simulink model "FullCarModelSim"  (R2018a)
settings: Solver=VariableStepAuto  StartTime=0.0  StopTime=8  FixedStep=0.001  MaxStep=0.002  MinStep=0.001  RelTol=1e-3  EnableMultiTasking=on
undefined symbols (not defined in the file): a, b, cg_height, cla, cp, I_zz, LLTD, m, step_steer, track_width_f, track_width_r, weight_dist, X
settings Model: Creator=tonylu  LastModifiedBy=tlton
settings OptimizationCC: LifeSpan=inf
settings DebuggingCC: SFUnexpectedBacktrackingDiag=warning  SFNoUnconditionalDefaultTransitionDiag=warning  SFExecutionAtInitializationDiag=none
settings CodeAppCC: StateflowObjectComments=on
settings GRTTargetCC: TargetLangStandard=C89/C90 (ANSI)  GeneratePreprocessorConditionals=Disable all
settings ConfigComp: CovMetricSettings=dw  CovHtmlReporting=on  CovSaveCumulativeToWorkspaceVar=on  CovSaveSingleToWorkspaceVar=on  CovExternalEMLEnable=off

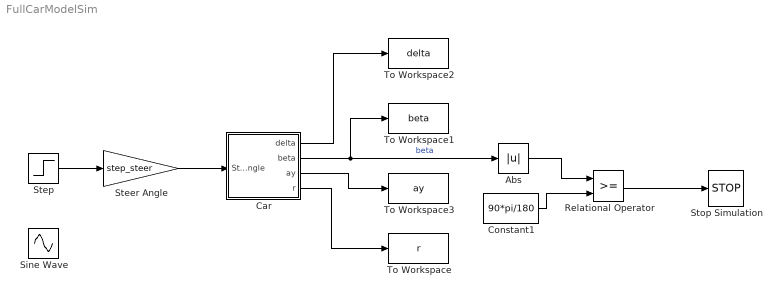
== system FullCarModelSim ==
  Abs : Abs
  Car : Subsystem
  Constant1 : Constant  Value=90*pi/180
  Relational Operator : RelationalOperator  OutDataTypeStr=boolean  RndMeth=Simplest
  Sine Wave : Sin  SampleTime=0
  Steer Angle : Gain  Gain=step_steer
  Step : Step  Time=0  SampleTime=0
  Stop Simulation : Stop
  To Workspace : ToWorkspace  VariableName=r  SaveFormat=Structure With Time  SampleTime=0.01
  To Workspace1 : ToWorkspace  VariableName=beta  SaveFormat=Structure With Time  SampleTime=0.01
  To Workspace2 : ToWorkspace  VariableName=delta  SaveFormat=Structure With Time  SampleTime=0.01
  To Workspace3 : ToWorkspace  VariableName=ay  SaveFormat=Structure With Time  SampleTime=0.01
  wires:
  Car/1(delta) -> To Workspace2/1
  Car/3(ay) -> To Workspace3/1
  Car/4(r) -> To Workspace/1
  Steer Angle/1 -> Car/1(Steer Angle)
  Car/2(beta) -> Abs/1, To Workspace1/1  "beta"
  Relational Operator/1 -> Stop Simulation/1
  Constant1/1 -> Relational Operator/2
  Abs/1 -> Relational Operator/1
  Step/1 -> Steer Angle/1

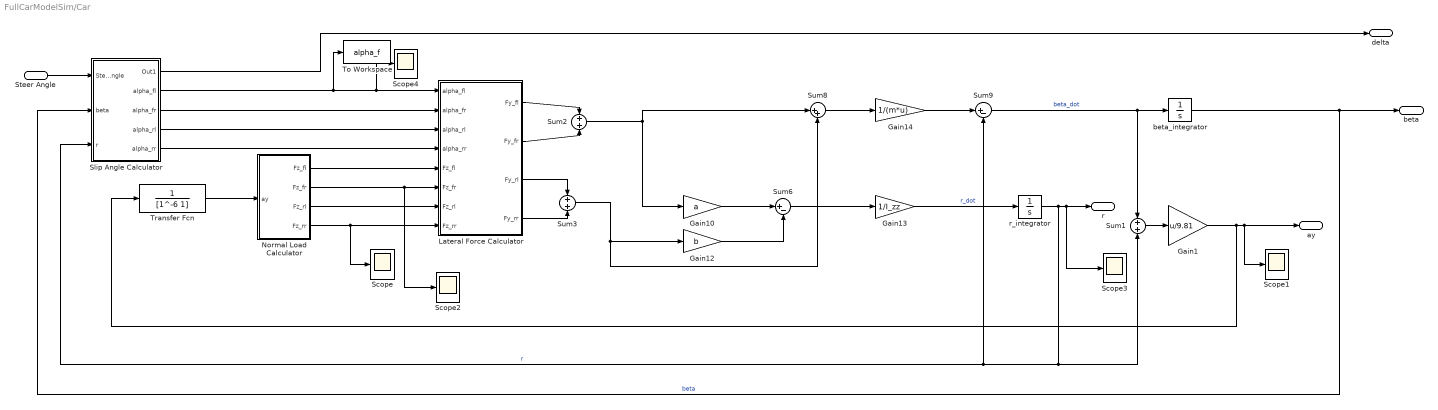
== system FullCarModelSim/Car ==
  Steer Angle : Inport
  Gain1 : Gain  Gain=u/9.81
  Gain10 : Gain  Gain=a
  Gain12 : Gain  Gain=b
  Gain13 : Gain  Gain=1/I_zz
  Gain14 : Gain  Gain=1/(m*u)
  Lateral Force Calculator : Subsystem
  Normal Load Calculator : Subsystem
  Scope{,1..4} (5 alike) : Scope
  Slip Angle Calculator : Subsystem
  Sum1 : Sum  Inputs=+|+
  Sum2 : Sum  Inputs=+|+
  Sum3 : Sum  Inputs=+|+
  Sum6 : Sum  Inputs=|+-
  Sum8 : Sum  Inputs=|++
  Sum9 : Sum  Inputs=|+-
  To Workspace : ToWorkspace  VariableName=alpha_f  SaveFormat=Structure With Time  SampleTime=0.01
  Transfer Fcn : TransferFcn  Denominator=[1^-6 1]
  beta_integrator : Integrator
  r_integrator : Integrator
  delta : Outport
  beta : Outport  Port=2
  ay : Outport  Port=3
  r : Outport  Port=4
  wires:
  Gain10/1 -> Sum6/1
  Gain12/1 -> Sum6/2
  Sum6/1 -> Gain13/1
  Gain13/1 -> r_integrator/1  "r_dot"
  Sum8/1 -> Gain14/1
  Gain14/1 -> Sum9/1
  Sum1/1 -> Gain1/1
  Steer Angle/1 -> Slip Angle Calculator/1(Steer Angle)
  Slip Angle Calculator/1(Out1) -> delta/1
  Slip Angle Calculator/2(alpha_fl) -> To Workspace/1, Scope4/1, Lateral Force Calculator/1(alpha_fl)
  Slip Angle Calculator/3(alpha_fr) -> Lateral Force Calculator/2(alpha_fr)
  Sum9/1 -> beta_integrator/1, Sum1/1  "beta_dot"
  beta_integrator/1 -> beta/1, Slip Angle Calculator/2(beta)  "beta"
  r_integrator/1 -> Slip Angle Calculator/3(r), Sum9/2, Sum1/2, Scope3/1, r/1  "r"
  Slip Angle Calculator/4(alpha_rl) -> Lateral Force Calculator/3(alpha_rl)
  Slip Angle Calculator/5(alpha_rr) -> Lateral Force Calculator/4(alpha_rr)
  Normal Load Calculator/1(Fz_fl) -> Lateral Force Calculator/5(Fz_fl)
  Normal Load Calculator/3(Fz_rl) -> Lateral Force Calculator/7(Fz_rl)
  Lateral Force Calculator/2(Fy_fr) -> Sum2/2
  Lateral Force Calculator/1(Fy_fl) -> Sum2/1
  Sum2/1 -> Gain10/1, Sum8/1
  Lateral Force Calculator/3(Fy_rl) -> Sum3/1
  Lateral Force Calculator/4(Fy_rr) -> Sum3/2
  Sum3/1 -> Sum8/2, Gain12/1
  Gain1/1 -> Transfer Fcn/1, Scope1/1, ay/1
  Normal Load Calculator/4("Fz_rr ") -> Scope/1, Lateral Force Calculator/8(Fz_rr)
  Normal Load Calculator/2(Fz_fr) -> Scope2/1, Lateral Force Calculator/6(Fz_fr)
  Transfer Fcn/1 -> Normal Load Calculator/1(ay)

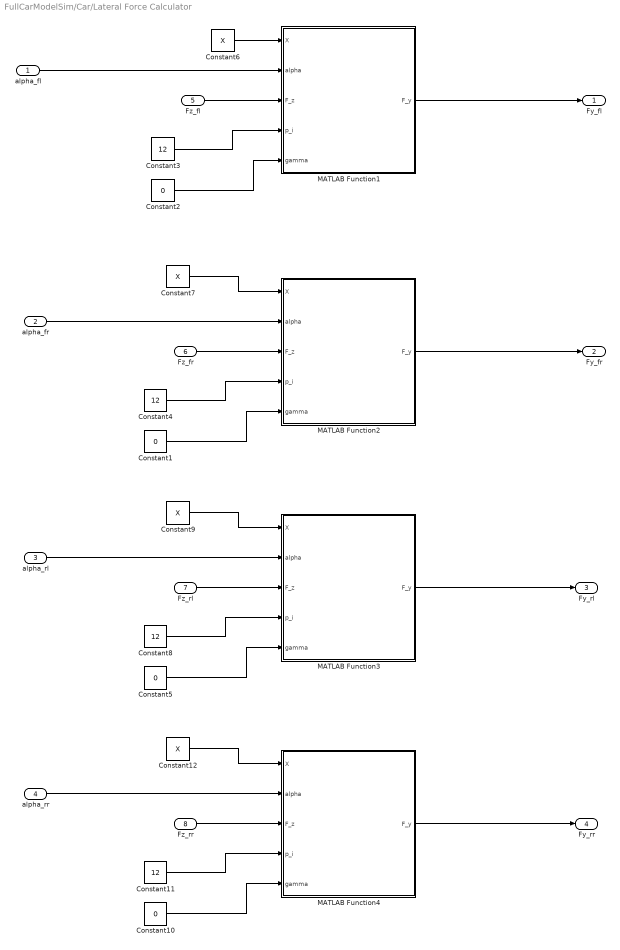
== system FullCarModelSim/Car/Lateral Force Calculator ==
  alpha_fl : Inport
  alpha_fr : Inport  Port=2
  alpha_rl : Inport  Port=3
  alpha_rr : Inport  Port=4
  Fz_fl : Inport  Port=5
  Fz_fr : Inport  Port=6
  Fz_rl : Inport  Port=7
  Fz_rr : Inport  Port=8
  Constant{1..2,5,10} (4 alike) : Constant  Value=0
  Constant{3..4,8,11} (4 alike) : Constant  Value=12
  Constant{6..7,9,12} (4 alike) : Constant  Value=X
  MATLAB Function1 : MATLAB Function  TreatAsAtomicUnit=on
  MATLAB Function2 : MATLAB Function  TreatAsAtomicUnit=on
  MATLAB Function3 : MATLAB Function  TreatAsAtomicUnit=on
  MATLAB Function4 : MATLAB Function  TreatAsAtomicUnit=on
  Fy_fl : Outport
  Fy_fr : Outport  Port=2
  Fy_rl : Outport  Port=3
  Fy_rr : Outport  Port=4
  wires:
  MATLAB Function2/1(F_y) -> Fy_fr/1
  Fz_fl/1 -> MATLAB Function1/3(F_z)
  Constant3/1 -> MATLAB Function1/4(p_i)
  Fz_fr/1 -> MATLAB Function2/3(F_z)
  MATLAB Function1/1(F_y) -> Fy_fl/1
  alpha_fr/1 -> MATLAB Function2/2(alpha)
  alpha_fl/1 -> MATLAB Function1/2(alpha)
  Constant4/1 -> MATLAB Function2/4(p_i)
  Constant2/1 -> MATLAB Function1/5(gamma)
  Constant7/1 -> MATLAB Function2/1(X)
  Constant6/1 -> MATLAB Function1/1(X)
  Constant1/1 -> MATLAB Function2/5(gamma)
  MATLAB Function3/1(F_y) -> Fy_rl/1
  Constant5/1 -> MATLAB Function3/5(gamma)
  alpha_rl/1 -> MATLAB Function3/2(alpha)
  Constant9/1 -> MATLAB Function3/1(X)
  Constant8/1 -> MATLAB Function3/4(p_i)
  Fz_rl/1 -> MATLAB Function3/3(F_z)
  MATLAB Function4/1(F_y) -> Fy_rr/1
  Constant10/1 -> MATLAB Function4/5(gamma)
  alpha_rr/1 -> MATLAB Function4/2(alpha)
  Constant12/1 -> MATLAB Function4/1(X)
  Constant11/1 -> MATLAB Function4/4(p_i)
  Fz_rr/1 -> MATLAB Function4/3(F_z)

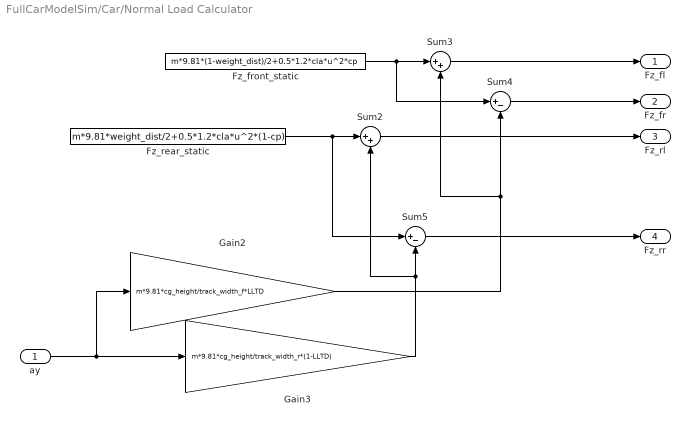
== system FullCarModelSim/Car/Normal Load Calculator ==
  ay : Inport
  Fz_front_static : Constant  Value=m*9.81*(1-weight_dist)/2+0.5*1.2*cla*u^2*cp
  Fz_rear_static : Constant  Value=m*9.81*weight_dist/2+0.5*1.2*cla*u^2*(1-cp)
  Gain2 : Gain  Gain=m*9.81*cg_height/track_width_f*LLTD
  Gain3 : Gain  Gain=m*9.81*cg_height/track_width_r*(1-LLTD)
  Sum2 : Sum  Inputs=|++
  Sum3 : Sum  Inputs=|++
  Sum4 : Sum  Inputs=|+-
  Sum5 : Sum  Inputs=|+-
  Fz_fl : Outport
  Fz_fr : Outport  Port=2
  Fz_rl : Outport  Port=3
  "Fz_rr " : Outport  Port=4
  wires:
  Sum4/1 -> Fz_fr/1
  Sum5/1 -> "Fz_rr "/1
  Fz_front_static/1 -> Sum4/1, Sum3/1
  Fz_rear_static/1 -> Sum5/1, Sum2/1
  Sum2/1 -> Fz_rl/1
  Gain3/1 -> Sum2/2, Sum5/2
  Sum3/1 -> Fz_fl/1
  ay/1 -> Gain2/1, Gain3/1
  Gain2/1 -> Sum4/2, Sum3/2

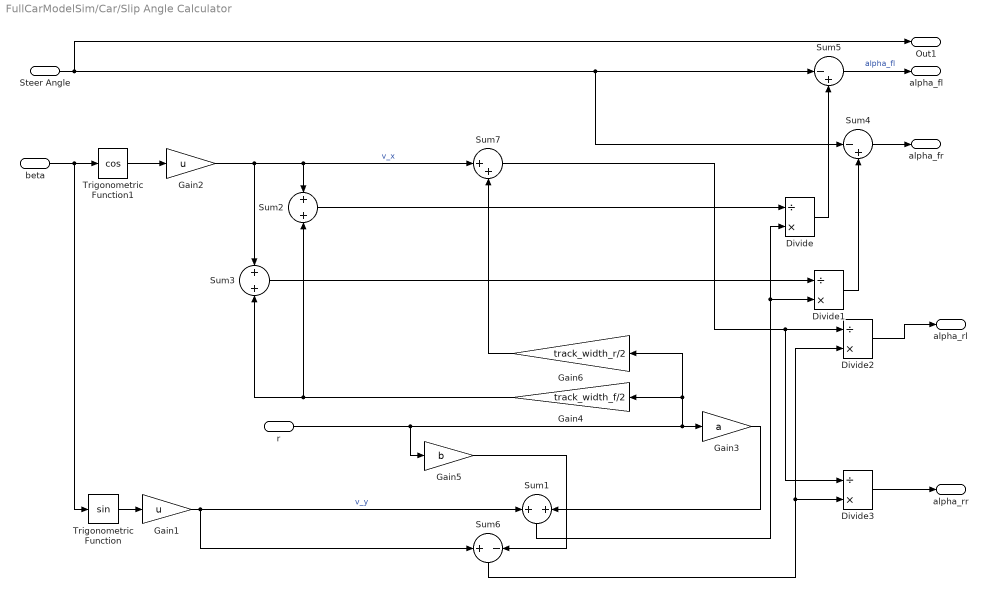
== system FullCarModelSim/Car/Slip Angle Calculator ==
  Steer Angle : Inport
  beta : Inport  Port=2
  r : Inport  Port=3
  Divide{,1..3} (4 alike) : Product  Inputs=/*
  Gain1 : Gain  Gain=u
  Gain2 : Gain  Gain=u
  Gain3 : Gain  Gain=a
  Gain4 : Gain  Gain=track_width_f/2
  Gain5 : Gain  Gain=b
  Gain6 : Gain  Gain=track_width_r/2
  Sum1 : Sum  Inputs=+|+
  Sum2 : Sum  Inputs=+|+
  Sum3 : Sum  Inputs=+|+
  Sum4 : Sum  Inputs=|-+
  Sum5 : Sum  Inputs=|-+
  Sum6 : Sum  Inputs=+|-
  Sum7 : Sum  Inputs=|++
  Trigonometric Function : Trigonometry
  Trigonometric Function1 : Trigonometry  Operator=cos
  Out1 : Outport
  alpha_fl : Outport  Port=2
  alpha_fr : Outport  Port=3
  alpha_rl : Outport  Port=4
  alpha_rr : Outport  Port=5
  wires:
  Sum5/1 -> alpha_fl/1  "alpha_fl"
  Trigonometric Function/1 -> Gain1/1
  Gain3/1 -> Sum1/2
  Divide/1 -> Sum5/2
  Sum3/1 -> Divide1/1
  Divide1/1 -> Sum4/2
  Sum4/1 -> alpha_fr/1
  Gain5/1 -> Sum6/2
  Sum2/1 -> Divide/1
  Divide2/1 -> alpha_rl/1
  Gain6/1 -> Sum7/2
  Divide3/1 -> alpha_rr/1
  Sum7/1 -> Divide3/1, Divide2/1
  Sum6/1 -> Divide3/2, Divide2/2
  Gain4/1 -> Sum3/2, Sum2/2
  Sum1/1 -> Divide1/2, Divide/2
  Gain1/1 -> Sum6/1, Sum1/1  "v_y"
  Gain2/1 -> Sum7/1, Sum2/1, Sum3/1  "v_x"
  Steer Angle/1 -> Sum4/1, Sum5/1, Out1/1
  r/1 -> Gain5/1, Gain6/1, Gain4/1, Gain3/1
  Trigonometric Function1/1 -> Gain2/1
  beta/1 -> Trigonometric Function/1, Trigonometric Function1/1

== matlab function FullCarModelSim/Car/Lateral Force Calculator/MATLAB Function1 ==
  data: X input; F_y output; alpha input; F_z input; p_i input; gamma input
function F_y  = lateralforce_pure(X,alpha,F_z,p_i,gamma)
%% Inputs
F_z = F_z/4.44822; % N to lbf

F_z0 = 200*ones(size(F_z)); %nominal load
p_i0 = 13*ones(size(p_i)); %nominal pressure

F_z = abs(F_z);

df_z = (F_z- F_z0)./F_z;
dp_i = (p_i-p_i0)./p_i;

%% Parameters

p_cy1 = X(1);
p_dy1 = X(2);
p_dy2 = X(3);
p_dy3 = X(4);
p_ey1 = X(5);
p_ey2 = X(6);
p_ey3 = X(7);
p_ey4 = X(8);
p_ey5 = X(9);
p_hy1 = X(10);
p_hy2 = X(11);
p_ky1 = X(12);
p_ky2 = X(13);
p_ky3 = X(14);
p_ky4 = X(15);
p_ky5 = X(16);
p_ky6 = X(17);
p_ky7 = X(18);
p_py1 = X(19);
p_py2 = X(20);
p_py3 = X(21);
p_py4 = X(22);
p_py5 = X(23);
p_vy1 = X(24);
p_vy2 = X(25);
p_vy3 = X(26);
p_vy4 = X(27);

%p_ey3 = 0
%p_dy1 = 1.8;
%p_dy2 = -0.05;

lambda_cy = 1;       % shape factor   
lambda_ey = 1;       % curvature 
lambda_hy = 0;       % horizontal shift
lambda_kyalpha = 1;  % cornering stiffness
lambda_kygamma = 1;  % camber force stiffness
lambda_muy = 0.55;      % peak friction coefficient
lambda_vy = 0;       % vertical shift

%%  Magic Formula Equations

K_yalpha = p_ky1.*F_z0.*(1+p_py1.*dp_i).*sin(p_ky4.*atan(F_z./...
    ((p_ky2 + p_ky5*gamma.^2).*(1+p_py2*dp_i).*F_z0))).*...
    (1-p_ky3.*abs(gamma)).*lambda_kyalpha;
K_ygamma = (p_ky6+p_ky7.*df_z).*(1+p_py5.*dp_i).*F_z.*lambda_kygamma;
S_vy0 = F_z.*(p_vy1+p_vy2.*df_z).*lambda_vy.*lambda_muy;
S_vygamma = F_z.*(p_vy3+p_vy4.*df_z).*gamma.*lambda_kygamma.*lambda_muy;
S_vy = S_vy0+S_vygamma;
S_hy0 = (p_hy1+p_hy2.*df_z).*lambda_hy;
S_hygamma = (K_ygamma.*gamma-S_vygamma)./K_yalpha;
S_hy = S_hy0+S_hygamma;
alpha_y = alpha+S_hy;
mu_y = (p_dy1+p_dy2.*df_z).*(1-p_dy3.*gamma.^2).*...
    (1+p_py3.*dp_i+p_py4.*dp_i.^2).*lambda_muy;
C_y = p_cy1.*lambda_cy;
D_y = mu_y.*F_z;
E_y = (p_ey1+p_ey2.*df_z).*(1+p_ey5.*gamma.^2-(p_ey3+p_ey4.*gamma).*sign(alpha_y)).*lambda_ey;
B_y = K_yalpha./C_y./D_y;

%Lateral Force
F_y = transpose(D_y.*sin(C_y.*atan(B_y.*alpha_y-E_y.*(B_y.*alpha_y-atan(B_y.*alpha_y))))+S_vy);

F_y = F_y*4.44822; % lbf to N

%F_y = -136*4.448*180/pi/2*alpha_y;

%F_y(F_z==0) = 0; %zero load

%F_y = K_yalpha*-0.0174533;

%F_y = -D_y

%F_y = mu_y;

end

== matlab function FullCarModelSim/Car/Lateral Force Calculator/MATLAB Function2 ==
  data: X input; F_y output; alpha input; F_z input; p_i input; gamma input
function F_y  = lateralforce_pure(X,alpha,F_z,p_i,gamma)
%% Inputs
F_z = F_z/4.44822; % N to lbf

F_z0 = 200*ones(size(F_z)); %nominal load
p_i0 = 13*ones(size(p_i)); %nominal pressure

F_z = abs(F_z);

df_z = (F_z- F_z0)./F_z;
dp_i = (p_i-p_i0)./p_i;

%% Parameters

p_cy1 = X(1);
p_dy1 = X(2);
p_dy2 = X(3);
p_dy3 = X(4);
p_ey1 = X(5);
p_ey2 = X(6);
p_ey3 = X(7);
p_ey4 = X(8);
p_ey5 = X(9);
p_hy1 = X(10);
p_hy2 = X(11);
p_ky1 = X(12);
p_ky2 = X(13);
p_ky3 = X(14);
p_ky4 = X(15);
p_ky5 = X(16);
p_ky6 = X(17);
p_ky7 = X(18);
p_py1 = X(19);
p_py2 = X(20);
p_py3 = X(21);
p_py4 = X(22);
p_py5 = X(23);
p_vy1 = X(24);
p_vy2 = X(25);
p_vy3 = X(26);
p_vy4 = X(27);

%p_ey3 = 0
%p_dy1 = 1.8;
%p_dy2 = -0.05;

lambda_cy = 1;       % shape factor   
lambda_ey = 1;       % curvature 
lambda_hy = 0;       % horizontal shift
lambda_kyalpha = 1;  % cornering stiffness
lambda_kygamma = 1;  % camber force stiffness
lambda_muy = 0.55;      % peak friction coefficient
lambda_vy = 0;       % vertical shift

%%  Magic Formula Equations

K_yalpha = p_ky1.*F_z0.*(1+p_py1.*dp_i).*sin(p_ky4.*atan(F_z./...
    ((p_ky2 + p_ky5*gamma.^2).*(1+p_py2*dp_i).*F_z0))).*...
    (1-p_ky3.*abs(gamma)).*lambda_kyalpha;
K_ygamma = (p_ky6+p_ky7.*df_z).*(1+p_py5.*dp_i).*F_z.*lambda_kygamma;
S_vy0 = F_z.*(p_vy1+p_vy2.*df_z).*lambda_vy.*lambda_muy;
S_vygamma = F_z.*(p_vy3+p_vy4.*df_z).*gamma.*lambda_kygamma.*lambda_muy;
S_vy = S_vy0+S_vygamma;
S_hy0 = (p_hy1+p_hy2.*df_z).*lambda_hy;
S_hygamma = (K_ygamma.*gamma-S_vygamma)./K_yalpha;
S_hy = S_hy0+S_hygamma;
alpha_y = alpha+S_hy;
mu_y = (p_dy1+p_dy2.*df_z).*(1-p_dy3.*gamma.^2).*...
    (1+p_py3.*dp_i+p_py4.*dp_i.^2).*lambda_muy;
C_y = p_cy1.*lambda_cy;
D_y = mu_y.*F_z;
E_y = (p_ey1+p_ey2.*df_z).*(1+p_ey5.*gamma.^2-(p_ey3+p_ey4.*gamma).*sign(alpha_y)).*lambda_ey;
B_y = K_yalpha./C_y./D_y;

%Lateral Force
F_y = transpose(D_y.*sin(C_y.*atan(B_y.*alpha_y-E_y.*(B_y.*alpha_y-atan(B_y.*alpha_y))))+S_vy);

F_y = F_y*4.44822; % lbf to N

%F_y = -136*4.448*180/pi/2*alpha_y;

%F_y(F_z==0) = 0; %zero load

%F_y = K_yalpha*-0.0174533;

%F_y = -D_y

%F_y = mu_y;

end

== matlab function FullCarModelSim/Car/Lateral Force Calculator/MATLAB Function3 ==
  data: X input; F_y output; alpha input; F_z input; p_i input; gamma input
function F_y  = lateralforce_pure(X,alpha,F_z,p_i,gamma)
%% Inputs
F_z = F_z/4.44822; % N to lbf

F_z0 = 200*ones(size(F_z)); %nominal load
p_i0 = 13*ones(size(p_i)); %nominal pressure

F_z = abs(F_z);

df_z = (F_z- F_z0)./F_z;
dp_i = (p_i-p_i0)./p_i;

%% Parameters

p_cy1 = X(1);
p_dy1 = X(2);
p_dy2 = X(3);
p_dy3 = X(4);
p_ey1 = X(5);
p_ey2 = X(6);
p_ey3 = X(7);
p_ey4 = X(8);
p_ey5 = X(9);
p_hy1 = X(10);
p_hy2 = X(11);
p_ky1 = X(12);
p_ky2 = X(13);
p_ky3 = X(14);
p_ky4 = X(15);
p_ky5 = X(16);
p_ky6 = X(17);
p_ky7 = X(18);
p_py1 = X(19);
p_py2 = X(20);
p_py3 = X(21);
p_py4 = X(22);
p_py5 = X(23);
p_vy1 = X(24);
p_vy2 = X(25);
p_vy3 = X(26);
p_vy4 = X(27);

%p_ey3 = 0
%p_dy1 = 1.8;
%p_dy2 = -0.05;

lambda_cy = 1;       % shape factor   
lambda_ey = 1;       % curvature 
lambda_hy = 0;       % horizontal shift
lambda_kyalpha = 1;  % cornering stiffness
lambda_kygamma = 1;  % camber force stiffness
lambda_muy = 0.55;      % peak friction coefficient
lambda_vy = 0;       % vertical shift

%%  Magic Formula Equations

K_yalpha = p_ky1.*F_z0.*(1+p_py1.*dp_i).*sin(p_ky4.*atan(F_z./...
    ((p_ky2 + p_ky5*gamma.^2).*(1+p_py2*dp_i).*F_z0))).*...
    (1-p_ky3.*abs(gamma)).*lambda_kyalpha;
K_ygamma = (p_ky6+p_ky7.*df_z).*(1+p_py5.*dp_i).*F_z.*lambda_kygamma;
S_vy0 = F_z.*(p_vy1+p_vy2.*df_z).*lambda_vy.*lambda_muy;
S_vygamma = F_z.*(p_vy3+p_vy4.*df_z).*gamma.*lambda_kygamma.*lambda_muy;
S_vy = S_vy0+S_vygamma;
S_hy0 = (p_hy1+p_hy2.*df_z).*lambda_hy;
S_hygamma = (K_ygamma.*gamma-S_vygamma)./K_yalpha;
S_hy = S_hy0+S_hygamma;
alpha_y = alpha+S_hy;
mu_y = (p_dy1+p_dy2.*df_z).*(1-p_dy3.*gamma.^2).*...
    (1+p_py3.*dp_i+p_py4.*dp_i.^2).*lambda_muy;
C_y = p_cy1.*lambda_cy;
D_y = mu_y.*F_z;
E_y = (p_ey1+p_ey2.*df_z).*(1+p_ey5.*gamma.^2-(p_ey3+p_ey4.*gamma).*sign(alpha_y)).*lambda_ey;
B_y = K_yalpha./C_y./D_y;

%Lateral Force
F_y = transpose(D_y.*sin(C_y.*atan(B_y.*alpha_y-E_y.*(B_y.*alpha_y-atan(B_y.*alpha_y))))+S_vy);

F_y = F_y*4.44822; % lbf to N

%F_y = -136*4.448*180/pi/2*alpha_y;

%F_y(F_z==0) = 0; %zero load

%F_y = K_yalpha*-0.0174533;

%F_y = -D_y

%F_y = mu_y;

end

== matlab function FullCarModelSim/Car/Lateral Force Calculator/MATLAB Function4 ==
  data: X input; F_y output; alpha input; F_z input; p_i input; gamma input
function F_y  = lateralforce_pure(X,alpha,F_z,p_i,gamma)
%% Inputs
F_z = F_z/4.44822; % N to lbf

F_z0 = 200*ones(size(F_z)); %nominal load
p_i0 = 13*ones(size(p_i)); %nominal pressure

F_z = abs(F_z);

df_z = (F_z- F_z0)./F_z;
dp_i = (p_i-p_i0)./p_i;

%% Parameters

p_cy1 = X(1);
p_dy1 = X(2);
p_dy2 = X(3);
p_dy3 = X(4);
p_ey1 = X(5);
p_ey2 = X(6);
p_ey3 = X(7);
p_ey4 = X(8);
p_ey5 = X(9);
p_hy1 = X(10);
p_hy2 = X(11);
p_ky1 = X(12);
p_ky2 = X(13);
p_ky3 = X(14);
p_ky4 = X(15);
p_ky5 = X(16);
p_ky6 = X(17);
p_ky7 = X(18);
p_py1 = X(19);
p_py2 = X(20);
p_py3 = X(21);
p_py4 = X(22);
p_py5 = X(23);
p_vy1 = X(24);
p_vy2 = X(25);
p_vy3 = X(26);
p_vy4 = X(27);

%p_ey3 = 0
%p_dy1 = 1.8;
%p_dy2 = -0.05;

lambda_cy = 1;       % shape factor   
lambda_ey = 1;       % curvature 
lambda_hy = 0;       % horizontal shift
lambda_kyalpha = 1;  % cornering stiffness
lambda_kygamma = 1;  % camber force stiffness
lambda_muy = 0.55;      % peak friction coefficient
lambda_vy = 0;       % vertical shift

%%  Magic Formula Equations

K_yalpha = p_ky1.*F_z0.*(1+p_py1.*dp_i).*sin(p_ky4.*atan(F_z./...
    ((p_ky2 + p_ky5*gamma.^2).*(1+p_py2*dp_i).*F_z0))).*...
    (1-p_ky3.*abs(gamma)).*lambda_kyalpha;
K_ygamma = (p_ky6+p_ky7.*df_z).*(1+p_py5.*dp_i).*F_z.*lambda_kygamma;
S_vy0 = F_z.*(p_vy1+p_vy2.*df_z).*lambda_vy.*lambda_muy;
S_vygamma = F_z.*(p_vy3+p_vy4.*df_z).*gamma.*lambda_kygamma.*lambda_muy;
S_vy = S_vy0+S_vygamma;
S_hy0 = (p_hy1+p_hy2.*df_z).*lambda_hy;
S_hygamma = (K_ygamma.*gamma-S_vygamma)./K_yalpha;
S_hy = S_hy0+S_hygamma;
alpha_y = alpha+S_hy;
mu_y = (p_dy1+p_dy2.*df_z).*(1-p_dy3.*gamma.^2).*...
    (1+p_py3.*dp_i+p_py4.*dp_i.^2).*lambda_muy;
C_y = p_cy1.*lambda_cy;
D_y = mu_y.*F_z;
E_y = (p_ey1+p_ey2.*df_z).*(1+p_ey5.*gamma.^2-(p_ey3+p_ey4.*gamma).*sign(alpha_y)).*lambda_ey;
B_y = K_yalpha./C_y./D_y;

%Lateral Force
F_y = transpose(D_y.*sin(C_y.*atan(B_y.*alpha_y-E_y.*(B_y.*alpha_y-atan(B_y.*alpha_y))))+S_vy);

F_y = F_y*4.44822; % lbf to N

%F_y = -136*4.448*180/pi/2*alpha_y;

%F_y(F_z==0) = 0; %zero load

%F_y = K_yalpha*-0.0174533;

%F_y = -D_y

%F_y = mu_y;

end
